simulink model "BlackBox"  (Simulink 8.3)
settings: Solver=ode45  StartTime=0.0  StopTime=100.0  RelTol=1e-3
values from neighbouring files (symbols this model uses):
  Ts = 0.005    [test.m]
settings Model: Creator=roadgont  LastModifiedBy=felipe
settings DataIOCC: SignalLoggingSaveFormat=Dataset
settings DebuggingCC: FrameProcessingCompatibilityMsg=error
settings HardwareCC: TargetBitPerLong=64  TargetBitPerPointer=64  TargetLongLongMode=on  TargetIntDivRoundTo=Zero  TargetEndianess=LittleEndian  TargetWordSize=64  TargetHWDeviceType=MATLAB Host  ProdEqTarget=off
settings RTWCC: SystemTargetFile=rtwsfcn.tlc  PackageGeneratedCodeAndArtifacts=on  PackageName=CajaNegra  TemplateMakefile=rtwsfcn_default_tmf  Description=S-Function Target  ProcessScript=rtwsfcn_make_rtw_hook  TargetLang=C++
settings STFCustomTargetCC: ModelReferenceCompliant=off  CompOptLevelCompliant=on  GeneratePreprocessorConditionals=Disable all  MATLABClassNameForMDSCustomization=Simulink.SoftwareTarget.TargetSpecificTriggerConfigurationBase  SystemTargetFile=rtwsfcn.tlc
settings CustomProperty: Value=on
settings ConfigComp: CovMetricSettings=dw  CovHtmlReporting=on  CovSaveCumulativeToWorkspaceVar=on  CovSaveSingleToWorkspaceVar=on  CovModelRefEnable=Off  CovExternalEMLEnable=off

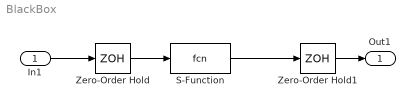
== system BlackBox ==
  In1 : Inport
  S-Function : S-Function  FunctionName=fcn  EnableBusSupport=off
  Zero-Order Hold : ZeroOrderHold  SampleTime=Ts
  Zero-Order Hold1 : ZeroOrderHold  SampleTime=Ts
  Out1 : Outport
  wires:
  Zero-Order Hold1/1 -> Out1/1
  In1/1 -> Zero-Order Hold/1
  Zero-Order Hold/1 -> S-Function/1
  S-Function/1 -> Zero-Order Hold1/1
